simulink model "Shaber_GearShiftStrategy"  (R2023b)
settings: Solver=FixedStepAuto  StartTime=0.0  StopTime=inf  FixedStep=0.001  RelTol=1e-3
PreLoadFcn:
  | load('ACS_1DModel23_Parameters_v2.mat');
undefined symbols (not defined in the file): AmbTemp, CellContCur, G_A, Init_SoC, kI, kP, nP, nS, SoCmin, ThrottleBP, TMaxMotor, VehicleMass
libraries: nesl_utility x21, fl_lib x14, sdl_lib x8, simulink x3, autolibrcnetworksystem x1, autolibmappedmotorcommon x1, autolibshared x1
(part 2 of 2)

== system Shaber_GearShiftStrategy/Chassis/Subsystem2 ==
  Ideal Rotational Motion Sensor : fl_lib/Mechanical/Mechanical Sensors/Ideal Rotational Motion Sensor  reference=foundation.enum.MeasurementReference.difference  acceleration_port=false  velocity_port=true  position_port=true  wrap_angle=simscape.enum.onoff.off  offset=0 rad
  Ideal Torque Sensor : fl_lib/Mechanical/Mechanical Sensors/Ideal Torque Sensor
  Mechanical Rotational Reference1 : fl_lib/Mechanical/Rotational Elements/Mechanical Rotational Reference
  PS-Simulink Converter : nesl_utility/PS-Simulink Converter  PhysicalDomain=network_engine_domain  SubClassName=ps_output  LeftPortType=input  RightPortType=output  PseudoPeriodic=off  Frequencies=[]  VectorFormat=1-D array  Unit=N*m  AffineConversion=off
  PS-Simulink Converter1 : nesl_utility/PS-Simulink Converter  PhysicalDomain=network_engine_domain  SubClassName=ps_output  LeftPortType=input  RightPortType=output  PseudoPeriodic=off  Frequencies=[]  VectorFormat=1-D array  Unit=rpm  AffineConversion=off
  PS-Simulink Converter2 : nesl_utility/PS-Simulink Converter  PhysicalDomain=network_engine_domain  SubClassName=ps_output  LeftPortType=input  RightPortType=output  PseudoPeriodic=off  Frequencies=[]  VectorFormat=1-D array  Unit=1  AffineConversion=off
  Terminator2 : Terminator
  Terminator3 : Terminator
  Conn1 : PMIOPort  Side=Right
  Conn2 : PMIOPort  Port=2  Side=Left
  FW Spd : Outport
  wires:
  PS-Simulink Converter/1 -> Terminator3/1  "WheelFrTq"
  PS-Simulink Converter2/1 -> Terminator2/1  "WheelFrAcc"
  PS-Simulink Converter1/1 -> FW Spd/1  "FWSpd [rpm]"
  connections:
  Ideal Torque Sensor/LConn1 -- Conn2/RConn1
  Conn1/RConn1 -- Ideal Torque Sensor/RConn1 -- Ideal Rotational Motion Sensor/LConn1
  Mechanical Rotational Reference1/LConn1 -- Ideal Rotational Motion Sensor/RConn1
  PS-Simulink Converter1/LConn1 -- Ideal Rotational Motion Sensor/RConn2
  PS-Simulink Converter/LConn1 -- Ideal Torque Sensor/RConn2
  Ideal Rotational Motion Sensor/RConn3 -- PS-Simulink Converter2/LConn1

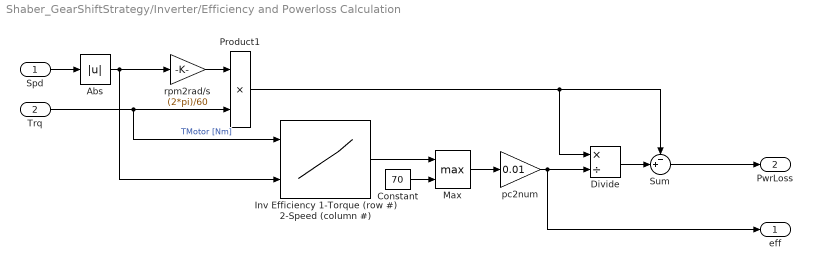
== system Shaber_GearShiftStrategy/Inverter/Efficiency and Powerloss Calculation ==
  Spd : Inport
  Trq : Inport  Port=2
  Abs : Abs  SaturateOnIntegerOverflow=off
  Constant : Constant  Value=70
  Divide : Product  Inputs=*/
  Inv Efficiency 1-Torque (row #) 2-Speed (column #) : Lookup_n-D  BreakpointsForDimension1=[-TMaxMotor TMaxMotor]  BreakpointsForDimension2=[0 7000]  Table=[0.8 0.9; 0.8 0.9]*100  InterpMethod=Cubic spline  ExtrapMethod=Cubic spline  InternalRulePriority=Speed  RndMeth=Simplest
      settings: InputPortMap=u0,u1
  Max : MinMax  Function=max  Inputs=2
  Product1 : Product
  Sum : Sum  Inputs=-+|
  pc2num : Gain  Gain=0.01
  rpm2rad/s : Gain  Gain=(2*pi)/60
  eff : Outport  VectorParamsAs1DForOutWhenUnconnected=off
  PwrLoss : Outport  Port=2  VectorParamsAs1DForOutWhenUnconnected=off
  wires:
  Product1/1 -> Sum/1, Divide/1
  Trq/1 -> Inv Efficiency 1-Torque (row #) 2-Speed (column #)/1, Product1/2  "TMotor [Nm]"
  Constant/1 -> Max/2
  Sum/1 -> PwrLoss/1
  Max/1 -> pc2num/1
  Divide/1 -> Sum/2
  rpm2rad/s/1 -> Product1/1
  Inv Efficiency 1-Torque (row #) 2-Speed (column #)/1 -> Max/1
  Spd/1 -> Abs/1
  Abs/1 -> rpm2rad/s/1, Inv Efficiency 1-Torque (row #) 2-Speed (column #)/2
  pc2num/1 -> Divide/2, eff/1

== system Shaber_GearShiftStrategy/Inverter/Transmission ==
  Abs1 : Abs  SaturateOnIntegerOverflow=off
  Constant : Constant  Value=2
  Data Type Conversion : DataTypeConversion  SaturateOnIntegerOverflow=off  RndMeth=Floor
  Relational Operator : RelationalOperator  Operator===  OutDataTypeStr=boolean  RndMeth=Simplest  InputSameDT=off
  Switch : Switch  Criteria=u2 > Threshold  SaturateOnIntegerOverflow=off  InputSameDT=off
  Transmission1 : Constant  Value=1*2.4*15/45
  Transmission2 : Constant  Value=1*1.5*15/45
  Transmission : Outport
  wires:
  [GearInd] -> Abs1/1
  Relational Operator/1 -> Data Type Conversion/1
  Transmission2/1 -> Switch/1
  Abs1/1 -> Relational Operator/2
  Switch/1 -> Transmission/1
  Constant/1 -> Relational Operator/1
  Transmission1/1 -> Switch/3
  Data Type Conversion/1 -> Switch/2

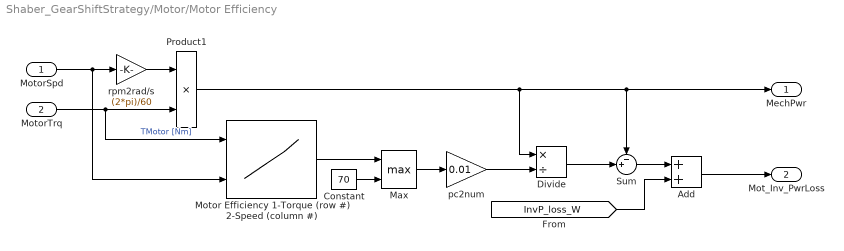
== system Shaber_GearShiftStrategy/Motor/Motor Efficiency ==
  MotorSpd : Inport
  MotorTrq : Inport  Port=2
  Add : Sum
  Constant : Constant  Value=70
  Divide : Product  Inputs=*/
  Max : MinMax  Function=max  Inputs=2
  Motor Efficiency 1-Torque (row #) 2-Speed (column #) : Lookup_n-D  BreakpointsForDimension1=[-TMaxMotor TMaxMotor]  BreakpointsForDimension2=[-7000 7000]  Table=[90 95; 90 95]  InterpMethod=Cubic spline  ExtrapMethod=Cubic spline  InternalRulePriority=Speed  RndMeth=Simplest
      settings: InputPortMap=u0,u1
  Product1 : Product
  Sum : Sum  Inputs=-+|
  pc2num : Gain  Gain=0.01
  rpm2rad/s : Gain  Gain=(2*pi)/60
  MechPwr : Outport  VectorParamsAs1DForOutWhenUnconnected=off
  Mot_Inv_PwrLoss : Outport  Port=2  VectorParamsAs1DForOutWhenUnconnected=off
  wires:
  Product1/1 -> MechPwr/1, Sum/1, Divide/1
  MotorTrq/1 -> Motor Efficiency 1-Torque (row #) 2-Speed (column #)/1, Product1/2  "TMotor [Nm]"
  Constant/1 -> Max/2
  Max/1 -> pc2num/1
  Divide/1 -> Sum/2
  rpm2rad/s/1 -> Product1/1
  MotorSpd/1 -> Motor Efficiency 1-Torque (row #) 2-Speed (column #)/2, rpm2rad/s/1
  Motor Efficiency 1-Torque (row #) 2-Speed (column #)/1 -> Max/1
  Sum/1 -> Add/1
  Add/1 -> Mot_Inv_PwrLoss/1
  [InvP_loss_W] -> Add/2
  pc2num/1 -> Divide/2

== system Shaber_GearShiftStrategy/Motor/Motor Time Constant (Response Smoothing) ==
  MaxT : Inport
  MotorTrqCmd : Inport  Port=2
  Divide2 : Product
  Gain : Gain  Gain=1/0.02
  Integrator : Integrator
  Interpolated Zero-crossing : Lookup_n-D  NumberOfTableDimensions=1  BreakpointsForDimension1=[-1 1]  Table=[-1 1]  ExtrapMethod=Clip  InternalRulePriority=Speed  RndMeth=Simplest
  Product1 : Product  Inputs=/*
  Sum : Sum  Inputs=|+-
  MotorTrq : Outport  InitialOutput=0  VectorParamsAs1DForOutWhenUnconnected=off
  wires:
  Sum/1 -> Integrator/1
  Gain/1 -> Product1/2, Sum/2
  Interpolated Zero-crossing/1 -> Divide2/2
  Integrator/1 -> Gain/1
  Divide2/1 -> MotorTrq/1
  MotorTrqCmd/1 -> Sum/1
  Product1/1 -> Interpolated Zero-crossing/1
  MaxT/1 -> Product1/1, Divide2/1

== system Shaber_GearShiftStrategy/Motor/Transmission ==
  Abs1 : Abs  SaturateOnIntegerOverflow=off
  Constant : Constant  Value=2
  Data Type Conversion : DataTypeConversion  SaturateOnIntegerOverflow=off  RndMeth=Floor
  Relational Operator : RelationalOperator  Operator===  OutDataTypeStr=boolean  RndMeth=Simplest  InputSameDT=off
  Switch : Switch  Criteria=u2 > Threshold  SaturateOnIntegerOverflow=off  InputSameDT=off
  Transmission1 : Constant  Value=1*2.4*15/45
  Transmission2 : Constant  Value=1*1.5*15/45
  Transmission : Outport
  wires:
  [GearInd] -> Abs1/1
  Relational Operator/1 -> Data Type Conversion/1
  Transmission2/1 -> Switch/1
  Abs1/1 -> Relational Operator/2
  Switch/1 -> Transmission/1
  Constant/1 -> Relational Operator/1
  Transmission1/1 -> Switch/3
  Data Type Conversion/1 -> Switch/2

== system Shaber_GearShiftStrategy/Rider/Subsystem1 ==
  Road Inclined (deg) : Inport
  Constant : Constant  Value=0
  Constant2 : Constant
  Display : Display
  Manual Switch : ManualSwitch
  Switch : Switch  Criteria=u2 > Threshold  SaturateOnIntegerOverflow=off  InputSameDT=off
  deg2rad : Gain  Gain=pi/180
  tag scope: RoadInclined=global
  wires:
  Manual Switch/1 -> Switch/1
  Constant/1 -> Manual Switch/2, Switch/3
  Switch/1 -> [RoadInclined]
  deg2rad/1 -> Display/1, Manual Switch/1  "rad"
  Constant2/1 -> Switch/2
  Road Inclined (deg)/1 -> deg2rad/1

== system Shaber_GearShiftStrategy/VSC/Checksum ==
  Torque_enable : Inport
  CurrentState : Inport  Port=2
  Driving State : Constant  Value=3
  Ignition State : Constant
  Logical Operator : Logic  AllPortsSameDT=off  OutDataTypeStr=boolean
  Logical Operator1 : Logic  AllPortsSameDT=off  OutDataTypeStr=boolean
  Logical Operator2 : Logic  AllPortsSameDT=off  OutDataTypeStr=boolean
  Out1 : Outport
  wires:
  Torque_enable/1 -> Logical Operator1/2
  Logical Operator2/1 -> Out1/1
  Ignition State/1 -> Logical Operator1/1
  CurrentState/1 -> Logical Operator/1
  Logical Operator/1 -> Logical Operator2/1
  Logical Operator1/1 -> Logical Operator2/2
  Driving State/1 -> Logical Operator/2

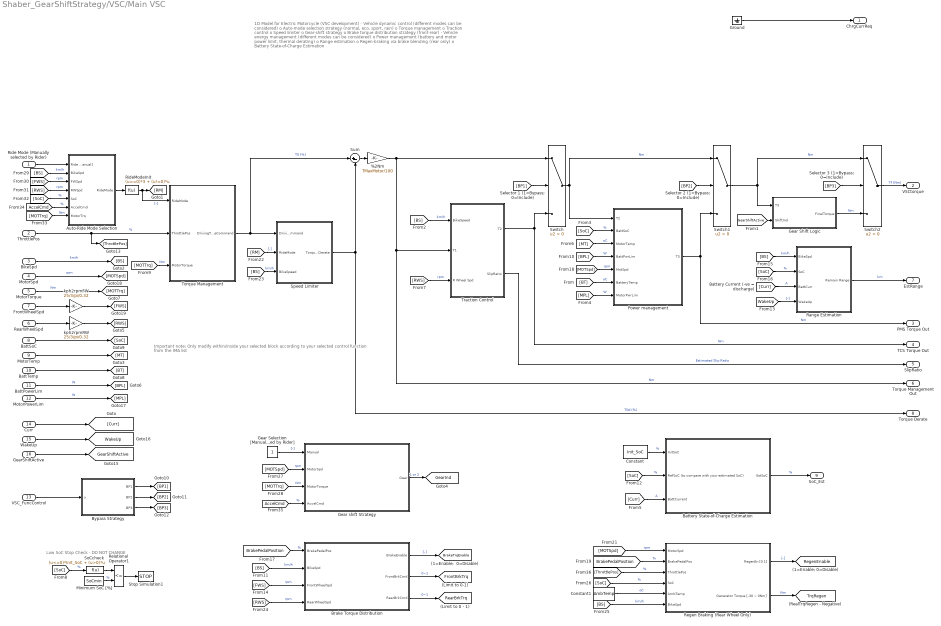
== system Shaber_GearShiftStrategy/VSC/Main VSC ==
  note: Low SoC Stop Check - DO NOT CHANGE
  note: 1D Model for Electric Motorcycle (VSC development)
      | · Vehicle dynamic control (different modes can be considered)
      | o Auto-mode selection strategy (normal, eco, sport, rain)
      | o Torque management
      | o Traction control
      | o Speed limiter
      | o Gear-shift strategy
      | o Brake torque distribution strategy (front-rear)
      | · Vehicle energy management (different modes can be considered)
      | o Power management (battery and motor power limit, thermal derating)
      | o Range estimation
      | o Regen-braking via brake blending (rear only)
      | o Battery State-of-Charge Estimation
  note: Important note:
      | Only modify within/inside your selected block according to your selected control function from the IMA list
  Ride Mode (Manually selected by Rider) : Inport
  ThrottlePos : Inport  Port=2
  BikeSpd : Inport  Port=3
  MotorSpd : Inport  Port=4
  MotorTorque : Inport  Port=5
  RearWheelSpd : Inport  Port=6
  FrontWheelSpd : Inport  Port=7
  BattSoC : Inport  Port=8
  MotorTemp : Inport  Port=9
  BattTemp : Inport  Port=10
  BattPowerLim : Inport  Port=11
  MotorPowerLim : Inport  Port=12
  VSC_FuncControl : Inport  Port=13
  Curr : Inport  Port=14
  WakeUp : Inport  Port=15
  GearShiftActive : Inport  Port=16
  %2Nm : Gain  Gain=TMaxMotor/100  OutDataTypeStr=Inherit: Same as input
  Auto-Ride Mode Selection : Subsystem
  Battery State-of-Charge Estimation : Subsystem
  Brake Torque Distribution : Subsystem
  Bypass Strategy : MATLAB Function  TreatAsAtomicUnit=on
  Constant : Constant  Value=Init_SoC
  Constant1 : Constant  Value=AmbTemp
  Gear Selection [Manually selected by Rider] : Constant
  Gear Shift Logic : Subsystem
  Gear shift Strategy : Subsystem
  Ground : Ground
  Minimum SoC [%] : Constant  Value=SoCmin
  Power management : Subsystem
  Range Estimation : Subsystem
  Regen Braking (Rear Wheel Only) : Subsystem
  Relational Operator1 : RelationalOperator  Operator=<=  OutDataTypeStr=boolean  RndMeth=Simplest  InputSameDT=off
  RideModeInit : Fcn  Expr=(u==0)*3 + (u!=0)*u
  SoCcheck : Fcn  Expr=(u<=0)*Init_SoC + (u>0)*u
  Speed Limiter : Subsystem
  Stop Simulation1 : Stop
  Sum : Sum  Inputs=|+-
  Switch : Switch  Criteria=u2 > Threshold  SaturateOnIntegerOverflow=off  InputSameDT=off
  Switch1 : Switch  Criteria=u2 > Threshold  SaturateOnIntegerOverflow=off  InputSameDT=off
  Switch2 : Switch  Criteria=u2 > Threshold  SaturateOnIntegerOverflow=off  InputSameDT=off
  Torque Management : Subsystem
  Traction Control : Subsystem
  kph2rpmFW : Gain  Gain=25/3/pi/0.32
  kph2rpmRW : Gain  Gain=25/3/pi/0.32
  ChrgCurrReq : Outport
  VSCtorque : Outport  Port=2
  PMS Torque Out : Outport  Port=3
  TCS Torque Out : Outport  Port=4
  SlipRatio : Outport  Port=5
  "Torque Management Out " : Outport  Port=6
  EstRange : Outport  Port=7
  Torque Derate : Outport  Port=8
  SoC_Est : Outport  Port=9
  tag scope: BrakeTrqEnable=global, FrontBrkTrq=global, GearInd=global, GearShiftActive=global, RearBrkTrq=global, RegenEnable=global, TrqRegen=global, WakeUp=global
  wires:
  Switch2/1 -> VSCtorque/1  "Tf (Nm)"
  [MOTSpd] -> Power management/5(MotSpd)  "rpm"
  BattPowerLim/1 -> [BPL]  "W"
  [BP2] -> Switch1/2
  BattSoC/1 -> [SoC]
  Bypass Strategy/1(BP1) -> [BP1]
  Ground/1 -> ChrgCurrReq/1
  RearWheelSpd/1 -> kph2rpmRW/1
  [BP3] -> Switch2/2
  FrontWheelSpd/1 -> kph2rpmFW/1
  [GearShiftActive] -> Gear Shift Logic/2(ShiftInd)
  [MPL] -> Power management/7(MotorPwrLim)  "W"
  BattTemp/1 -> [BT]
  [MT] -> Power management/3(MotorTemp)  "oC"
  Range Estimation/1(Remain Range) -> EstRange/1  "km"
  [BP1] -> Switch/2
  MotorPowerLim/1 -> [MPL]  "W"
  Traction Control/2(SlipRatio) -> SlipRatio/1  "Estimated Slip Ratio"
  [WakeUp] -> Range Estimation/4(WakeUp)  "[-]"
  Traction Control/1(T2) -> Switch/3, TCS Torque Out/1  "Nm"
  [Curr] -> Range Estimation/3(BattCurr)  "A"
  [BT] -> Power management/6(BatteryTemp)  "oC"
  GearShiftActive/1 -> [GearShiftActive]
  BikeSpd/1 -> [BS]  "km/h"
  ThrottlePos/1 -> [ThrottlePos], Torque Management/2(ThrottlePos)  "%"
  Power management/1(T3) -> PMS Torque Out/1, Switch1/3  "Nm"
  [BS] -> Range Estimation/1(BikeSpd)  "km/h"
  [SoC] -> Power management/2(BattSoC)  "%"
  [RWS] -> Traction Control/3(R Wheel Spd)  "rpm"
  kph2rpmRW/1 -> [RWS]
  kph2rpmFW/1 -> [FWS]
  Switch/1 -> Switch1/1, Power management/1(T2)  "Nm"
  [SoC] -> Range Estimation/2(SoC)  "%"
  VSC_FuncControl/1 -> Bypass Strategy/1(u)
  Switch1/1 -> Switch2/1, Gear Shift Logic/1(T3)  "Nm"
  MotorSpd/1 -> [MOTSpd]  "rpm"
  [BPL] -> Power management/4(BattPwrLim)  "W"
  Gear Shift Logic/1(FinalTorque) -> Switch2/3  "Nm"
  Curr/1 -> [Curr]
  RideModeInit/1 -> [RM], Torque Management/1(RideMode)  "[-]"
  Bypass Strategy/2(BP2) -> [BP2]
  WakeUp/1 -> [WakeUp]
  Bypass Strategy/3(BP3) -> [BP3]
  %2Nm/1 -> Switch/1, Traction Control/2(T1), "Torque Management Out "/1  "Nm"
  MotorTemp/1 -> [MT]
  Battery State-of-Charge Estimation/1(EstSoC) -> SoC_Est/1  "%"
  [Curr] -> Battery State-of-Charge Estimation/3(BattCurrent)  "A"
  Constant/1 -> Battery State-of-Charge Estimation/1(InitSoC)  "%"
  SoCcheck/1 -> Relational Operator1/1
  Minimum SoC [%]/1 -> Relational Operator1/2  "%"
  Relational Operator1/1 -> Stop Simulation1/1
  [SoC] -> SoCcheck/1  "%"
  Gear Selection [Manually selected by Rider]/1 -> Gear shift Strategy/1(Manual)  "[-]"
  Gear shift Strategy/1(Gear) -> [GearInd]  "1 or 2"
  MotorTorque/1 -> [MOTTrq]  "Nm"
  [MOTTrq] -> Torque Management/3(MotorTorque)  "Nm"
  [SoC] -> Battery State-of-Charge Estimation/2(RefSoC (to compare with your estimated SoC))  "%"
  Brake Torque Distribution/2(FrontBrkCmd) -> [FrontBrkTrq]  "0~1"
  Brake Torque Distribution/3(RearBrkCmd) -> [RearBrkTrq]  "0~1"
  [BrakePedalPosition] -> Brake Torque Distribution/1(BrakePedalPos)  "%"
  [BrakePedalPosition] -> Regen Braking (Rear Wheel Only)/2(BrakePedalPos)  "%"
  [ThrottlePos] -> Regen Braking (Rear Wheel Only)/3(ThrottlePos)  "%"
  Regen Braking (Rear Wheel Only)/1(RegenEn [0 1]) -> [RegenEnable]  "[-]"
  Regen Braking (Rear Wheel Only)/2(Generator Torque [-30 ~ 0Nm]) -> [TrqRegen]  "Nm"
  [MOTSpd] -> Regen Braking (Rear Wheel Only)/1(MotorSpd)  "rpm"
  Brake Torque Distribution/1(BrakeEnable) -> [BrakeTrqEnable]  "[-]"
  Sum/1 -> %2Nm/1
  Torque Management/1(DrivingTorqueCommand) -> Sum/1, Speed Limiter/1(DrivingTorqueCommand)  "T0 (%)"
  Speed Limiter/1("TorqueDerate ") -> Torque Derate/1, Sum/2  "T0d (%)"
  [RM] -> Speed Limiter/2(RideMode)  "[-]"
  [BS] -> Speed Limiter/3(BikeSpeed)  "km/h"
  [BS] -> Traction Control/1(BikeSpeed)  "km/h"
  [BS] -> Brake Torque Distribution/2(BikeSpd)  "km/h"
  [FWS] -> Brake Torque Distribution/3(FrontWheelSpd)  "rpm"
  [RWS] -> Brake Torque Distribution/4(RearWheelSpd)  "rpm"
  [BS] -> Regen Braking (Rear Wheel Only)/6(BikeSpd)  "km/h"
  [SoC] -> Regen Braking (Rear Wheel Only)/4(SoC)  "%"
  Constant1/1 -> Regen Braking (Rear Wheel Only)/5(AmbTemp)  "oC"
  [MOTSpd] -> Gear shift Strategy/2(MotorSpd)  "rpm"
  [MOTTrq] -> Gear shift Strategy/3(MotorTorque)  "Nm"
  [BS] -> Auto-Ride Mode Selection/2(BikeSpd)  "km/h"
  [FWS] -> Auto-Ride Mode Selection/3(FWSpd)  "rpm"
  [RWS] -> Auto-Ride Mode Selection/4(RWSpd)  "rpm"
  [SoC] -> Auto-Ride Mode Selection/5(SoC)  "%"
  [MOTTrq] -> Auto-Ride Mode Selection/7(MotorTrq)  "Nm"
  [AccelCmd] -> Auto-Ride Mode Selection/6(AccelCmd)  "%"
  [AccelCmd] -> Gear shift Strategy/4(AccelCmd)  "%"
  Ride Mode (Manually selected by Rider)/1 -> Auto-Ride Mode Selection/1(Ride Mode [Manual])
  Auto-Ride Mode Selection/1(RideMode) -> RideModeInit/1

== system Shaber_GearShiftStrategy/Chassis/2-Speeds CVT/Subsystem1 ==
  Ideal Rotational Motion Sensor : fl_lib/Mechanical/Mechanical Sensors/Ideal Rotational Motion Sensor  reference=foundation.enum.MeasurementReference.difference  acceleration_port=false  velocity_port=true  position_port=true  wrap_angle=simscape.enum.onoff.off  offset=0 rev
  Ideal Torque Sensor : fl_lib/Mechanical/Mechanical Sensors/Ideal Torque Sensor
  Mechanical Rotational Reference1 : fl_lib/Mechanical/Rotational Elements/Mechanical Rotational Reference
  PS-Simulink Converter : nesl_utility/PS-Simulink Converter  PhysicalDomain=network_engine_domain  SubClassName=ps_output  LeftPortType=input  RightPortType=output  PseudoPeriodic=off  Frequencies=[]  VectorFormat=1-D array  Unit=N*m  AffineConversion=off
  PS-Simulink Converter1 : nesl_utility/PS-Simulink Converter  PhysicalDomain=network_engine_domain  SubClassName=ps_output  LeftPortType=input  RightPortType=output  PseudoPeriodic=off  Frequencies=[]  VectorFormat=1-D array  Unit=rpm  AffineConversion=off
  PS-Simulink Converter2 : nesl_utility/PS-Simulink Converter  PhysicalDomain=network_engine_domain  SubClassName=ps_output  LeftPortType=input  RightPortType=output  PseudoPeriodic=off  Frequencies=[]  VectorFormat=1-D array  Unit=1  AffineConversion=off
  Terminator2 : Terminator
  Conn1 : PMIOPort  Side=Right
  Conn2 : PMIOPort  Port=2  Side=Left
  Spd : Outport
  Trq : Outport  Port=2
  wires:
  PS-Simulink Converter2/1 -> Terminator2/1  "OutShaftAcc"
  PS-Simulink Converter/1 -> Trq/1  "OutShaftTq"
  PS-Simulink Converter1/1 -> Spd/1  "OutShaftSpd(rpm)"
  connections:
  Ideal Rotational Motion Sensor/RConn3 -- PS-Simulink Converter2/LConn1
  PS-Simulink Converter/LConn1 -- Ideal Torque Sensor/RConn2
  PS-Simulink Converter1/LConn1 -- Ideal Rotational Motion Sensor/RConn2
  Mechanical Rotational Reference1/LConn1 -- Ideal Rotational Motion Sensor/RConn1
  Conn1/RConn1 -- Ideal Rotational Motion Sensor/LConn1 -- Ideal Torque Sensor/RConn1
  Ideal Torque Sensor/LConn1 -- Conn2/RConn1

== system Shaber_GearShiftStrategy/VSC/Main VSC/Auto-Ride Mode Selection ==
  note: To be replaced by your logic
  note: Ride Mode definition: 1 = Rain ; 2 = Eco ; 3 = Normal ; 4 = Sport
      |
      | Requirement:
      | - Develop a logic in Stateflow to decide the bike operational mode according to the update of system state (inputs available for this function)
      |
      | Example: Switch to Sport mode when having high AccelCmd
      |
      | Inputs:
      | - BikeSpd, FWSpd, RWSpd, SoC, AccelCmd, MotorTrq
  Ride Mode [Manual] : Inport
  BikeSpd : Inport  Port=2
  FWSpd : Inport  Port=3
  RWSpd : Inport  Port=4
  SoC : Inport  Port=5
  AccelCmd : Inport  Port=6
  MotorTrq : Inport  Port=7
  Constant : Constant  Value=0
  Ground : Ground
  Switch : Switch  Criteria=u2 > Threshold  SaturateOnIntegerOverflow=off  InputSameDT=off
  RideMode : Outport
  wires:
  Ride Mode [Manual]/1 -> Switch/3  "Manual"
  Switch/1 -> RideMode/1
  Constant/1 -> Switch/2
  Ground/1 -> Switch/1

== system Shaber_GearShiftStrategy/VSC/Main VSC/Battery State-of-Charge Estimation ==
  note: Requirement:
      | Create a logic to estimate the State of Charge of the battery:
      | - Use any input from the MainBus
      | - Build an Equivalent Circuit Model (ECM) using Simulink blocks (not using battery components in Simulink)
      | - Limit the SoC within 0 - 100%
      | - Employ the InitSoC input as the initial SoC of the battery (can be used to interpolate the Initial remained Capacity)
      |
      | Note: can get ECM parameters from the "Battery Pack" block
  InitSoC : Inport
  RefSoC (to compare with your estimated SoC) : Inport  Port=2
  BattCurrent : Inport  Port=3
  EstSoC : Outport

== system Shaber_GearShiftStrategy/VSC/Main VSC/Brake Torque Distribution ==
  note: BrakeEnable = 0: use default values defined from the model (Front/Rear = 20%/80% by default)
      | BrakeEnable = 1: use your own brake torque distribution
  note: Requirement:
      | Develop a controller to distribute the brake torque applied to the front and rear wheels (already added in the Chassis model) when applying Brake
      |
      | Note:
      | use any input from the Bus or elsewhere
      |
      | Example: some ideas about brake torque distribution from this link:
      |
      | https://www.drivingtests.co.nz/roadcode-questions/motorbike/motorbike-specific-questions/how-much-braking-comes-from-the-front-wh/
      |
      | https://www.lazymotorbike.eu/tips/braking/
  BrakePedalPos : Inport
  BikeSpd : Inport  Port=2
  FrontWheelSpd : Inport  Port=3
  RearWheelSpd : Inport  Port=4
  Ground : Ground
  Terminator : Terminator
  km/h 2 rpm : Gain  Gain=25/3/pi/0.32
  BrakeEnable : Outport
  FrontBrkCmd : Outport  Port=2
  RearBrkCmd : Outport  Port=3
  wires:
  Ground/1 -> BrakeEnable/1
  BikeSpd/1 -> km/h 2 rpm/1  "km/h"
  km/h 2 rpm/1 -> Terminator/1  "rpm"

== system Shaber_GearShiftStrategy/VSC/Main VSC/Gear Shift Logic ==
  note: Gear Shift Logic - DO NOT TOUCH
  T3 : Inport
  ShiftInd : Inport  Port=2
  Gear Shift Logic : Stateflow chart  TreatAsAtomicUnit=on
  Sum : Sum  Inputs=|+-
  FinalTorque : Outport
  wires:
  Gear Shift Logic/1(TqMod) -> Sum/2
  ShiftInd/1 -> Gear Shift Logic/2(ShiftInd)
  T3/1 -> Sum/1, Gear Shift Logic/1(T3)
  Sum/1 -> FinalTorque/1

== system Shaber_GearShiftStrategy/VSC/Main VSC/Gear shift Strategy ==
  note: Gear 1 ratio = 2.5 (speed reduction)
      | Gear 2 ratio = 4 (speed reduction)
      |
      | Requirement:
      | Develop a logic to switch between 2 speeds of the CVT transmission as shown in the Chassis model (can be expanded to more than 2 ratios). The logic could be based on vehicle speed, motor speed, Acceleration command, motor torque ...
      |
      | Example:
      | when high MotorTorque, Gear 2 can be used to increase Torque;
      | when high AccelCmd and low MotorTorque, Gear 1 can be used.
  Manual : Inport
  MotorSpd : Inport  Port=2
  MotorTorque : Inport  Port=3
  AccelCmd : Inport  Port=4
  Bus Selector : BusSelector  OutputSignals=RiderCmd.RiderMode
  Chart : Stateflow chart  TreatAsAtomicUnit=on
  Scope : Scope  NumInputPorts=3
  Gear : Outport
  wires:
  [BUS] -> Bus Selector/1
  AccelCmd/1 -> Chart/3(AccelCmd), Scope/2
  Bus Selector/1 -> Chart/4(RiderMode)  "<RiderMode>"
  Manual/1 -> Chart/1(Manual)
  Chart/1(Gear) -> Gear/1, Scope/3
  MotorSpd/1 -> Chart/2(MotorSpd), Scope/1

== system Shaber_GearShiftStrategy/VSC/Main VSC/Power management ==
  note: Requirement:
      | Develop the following logics:
      | - Battery power limit (using BattSoC, BattPwrLim)
      | - Motor power limit (using MotorPwrLim)
      | - Thermal derating (using MotorTemp and BatteryTemp)
      |
      | Note: T3 = T2 - T2d
      | BattPwrLim and MotorPwrLim are the maximum power available on Battery and Motor, respectively
      |
      | Example:
      | when high MotorTemp or BatteryTemp, Torque output will be derated
  T2 : Inport
  BattSoC : Inport  Port=2
  MotorTemp : Inport  Port=3
  BattPwrLim : Inport  Port=4
  MotSpd : Inport  Port=5
  BatteryTemp : Inport  Port=6
  MotorPwrLim : Inport  Port=7
  Ground : Ground
  Sum : Sum  Inputs=-+|
  T3 : Outport
  wires:
  T2/1 -> Sum/2
  Sum/1 -> T3/1
  Ground/1 -> Sum/1  "T2d (Nm)"

== system Shaber_GearShiftStrategy/VSC/Main VSC/Range Estimation ==
  BikeSpd : Inport
  SoC : Inport  Port=2
  BattCurr : Inport  Port=3
  WakeUp : Inport  Port=4
  AmbTemp : Constant  Value=AmbTemp
  Minimum Allowable Battery SoC [%] : Constant  Value=SoCmin
  Model Discrete Sample Time [s] : Constant  Value=0.01
  Range estimation : Subsystem
  SoCcheck : Fcn  Expr=(u<=0)*Init_SoC + (u>0)*u
  Theoretical Max. Range [km] : Constant  Value=150
  Typical Consumption Rate [%/km] : Constant  Value=0.625
  Remain Range : Outport
  wires:
  Range estimation/1(Ro) -> Remain Range/1  "km"
  Minimum Allowable Battery SoC [%]/1 -> Range estimation/4(SoCmin)  "%"
  AmbTemp/1 -> Range estimation/8(AmbTemp)  "oC"
  SoCcheck/1 -> Range estimation/5(SoC)  "%"
  BattCurr/1 -> Range estimation/7(BattCurr)  "A"
  SoC/1 -> SoCcheck/1
  Typical Consumption Rate [%/km]/1 -> Range estimation/6(AvgConR)  "%SoC/km"
  Model Discrete Sample Time [s]/1 -> Range estimation/2(dT)  "s"
  BikeSpd/1 -> Range estimation/1(BSpd)  "km/h"
  WakeUp/1 -> Range estimation/9(WakeUp)  "on/off"
  Theoretical Max. Range [km]/1 -> Range estimation/3(RMax)  "km"

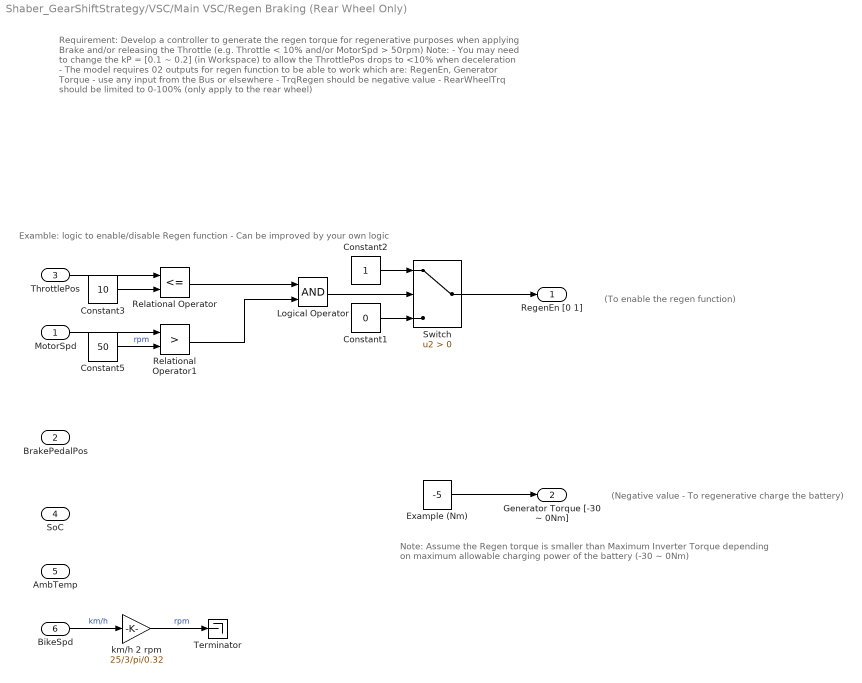
== system Shaber_GearShiftStrategy/VSC/Main VSC/Regen Braking (Rear Wheel Only) ==
  note: Examble: logic to enable/disable Regen function - Can be improved by your own logic
  note: (To enable the regen function)
  note: (Negative value - To regenerative charge the battery)
  note: Requirement:
      | Develop a controller to generate the regen torque for regenerative purposes when applying Brake and/or releasing the Throttle (e.g. Throttle < 10% and/or MotorSpd > 50rpm)
      |
      | Note:
      | - You may need to change the kP = [0.1 ~ 0.2] (in Workspace) to allow the ThrottlePos drops to <10% when deceleration
      | - The model requires 02 outputs for regen function to be able to work which are: RegenEn, Generator Torque
      | - use any input from the Bus or elsewhere
      | - TrqRegen should be negative value
      | - RearWheelTrq should be limited to 0-100% (only apply to the rear wheel)
  note: Note: Assume the Regen torque is smaller than Maximum Inverter Torque
      | depending on maximum allowable charging power of the battery
      | (-30 ~ 0Nm)
  MotorSpd : Inport
  BrakePedalPos : Inport  Port=2
  ThrottlePos : Inport  Port=3
  SoC : Inport  Port=4
  AmbTemp : Inport  Port=5
  BikeSpd : Inport  Port=6
  Constant1 : Constant  Value=0
  Constant2 : Constant
  Constant3 : Constant  Value=10
  Constant5 : Constant  Value=50
  Example (Nm) : Constant  Value=-5
  Logical Operator : Logic  AllPortsSameDT=off  OutDataTypeStr=boolean
  Relational Operator : RelationalOperator  Operator=<=  OutDataTypeStr=boolean  RndMeth=Simplest  InputSameDT=off
  Relational Operator1 : RelationalOperator  Operator=>  OutDataTypeStr=boolean  RndMeth=Simplest  InputSameDT=off
  Switch : Switch  Criteria=u2 > Threshold  SaturateOnIntegerOverflow=off  InputSameDT=off
  Terminator : Terminator
  km/h 2 rpm : Gain  Gain=25/3/pi/0.32
  RegenEn [0 1] : Outport
  Generator Torque [-30 ~ 0Nm] : Outport  Port=2
  wires:
  Example (Nm)/1 -> Generator Torque [-30 ~ 0Nm]/1
  Switch/1 -> RegenEn [0 1]/1
  Constant1/1 -> Switch/3
  Constant2/1 -> Switch/1
  Logical Operator/1 -> Switch/2
  ThrottlePos/1 -> Relational Operator/1
  Constant3/1 -> Relational Operator/2
  MotorSpd/1 -> Relational Operator1/1
  Constant5/1 -> Relational Operator1/2  "rpm"
  Relational Operator/1 -> Logical Operator/1
  Relational Operator1/1 -> Logical Operator/2
  km/h 2 rpm/1 -> Terminator/1  "rpm"
  BikeSpd/1 -> km/h 2 rpm/1  "km/h"

== system Shaber_GearShiftStrategy/VSC/Main VSC/Speed Limiter ==
  note: Fixed saturation - DO NOT CHANGE
  note: Requirement:
      | Create a closed-loop controller inside "Forward Torque Derater" block to ensure that the bike speed does not come out of range within its current operation mode, by considering:
      | Input: (you can use all or some of these available inputs: BikeSpeed, RideMode, TorqueDemand), more inputs can be collected from the Bus
      | Output: controlled TorqueDerate
      | Note: the logic inside "Forward Torque Derater" block is an example using open-loop control to generate the TorqueDerate
  DrivingTorqueCommand : Inport
  RideMode : Inport  Port=2
  BikeSpeed : Inport  Port=3
  Constant1 : Constant  Value=0
  Forward Torque Derater : Subsystem
  Saturation : Saturate  UpperLimit=TMaxMotor  LowerLimit=0
  Saturation Dynamic : simulink/Discontinuities/Saturation Dynamic  OutMin=[]  OutMax=[]  OutDataTypeStr=Inherit: Same as second input  OutDataType=fixdt(1, 16)  OutScaling=2^-10  DoSatur=off
  "TorqueDerate " : Outport
  wires:
  Saturation Dynamic/1 -> "TorqueDerate "/1  "T0d"
  RideMode/1 -> Forward Torque Derater/1(RideMode)
  BikeSpeed/1 -> Forward Torque Derater/2(BikeSpeed)  "km/h"
  Constant1/1 -> Saturation Dynamic/3
  Forward Torque Derater/1(TqMod) -> Saturation Dynamic/2
  DrivingTorqueCommand/1 -> Saturation/1
  Saturation/1 -> Saturation Dynamic/1

== system Shaber_GearShiftStrategy/VSC/Main VSC/Torque Management ==
  note: y is the Reference Torque for your closed-loop controller
  note: Fixed Open-loop Torque Map - DO NOT CHANGE or DELETE
  note: Requirement:
      |
      | Create a closed-loop controller to control the torque demand (TqDemand) to follow the desired torque (y) interpolated based on ThrottleBP position
      | - Use MotorTorque input as the actual torque feedback of the motor
      |
      | Note: in here we have an open-loop torque demand (y), which is linear interpolated based on the ThrottleBP and RideMode
  RideMode : Inport
  ThrottlePos : Inport  Port=2
  MotorTorque : Inport  Port=3
  Constant1 : Constant  Value=ThrottleBP  VectorParams1D=off
  Eco : Constant  Value=[0 0 0 4 8 13 16 20 25 30 35 40 45 48 50 55 60 65 70 75 80]'  VectorParams1D=off
  Linear interpolation : simulink/Lookup Tables/Lookup Table Dynamic  LookUpMeth=Interpolation-Use End Values  OutDataType=fixdt('double')  OutScaling=[]  OutputDataTypeScalingMode=Specify via dialog  OutDataTypeStr=double  DoSatur=off
  Multiport Switch : MultiPortSwitch  Inputs=4  DataPortForDefault=Additional data port  SaturateOnIntegerOverflow=off  InputSameDT=off
  Norm : Constant  Value=[0 0 0 5 10 15 20 28 35 40 45 50 55 60 65 70 80 85 90 95 100]'  VectorParams1D=off
  Rain : Constant  Value=[0 0 0 3 8 13 18 22 28 32 36 40 44 48 52 56 60 64 66 68 70]'  VectorParams1D=off
  Sport : Constant  Value=[0 0 0 5 15 20 25 30 40 50 55 60 65 75 80 90 95 100 100 100 100]'  VectorParams1D=off
  DrivingTorqueCommand : Outport
  wires:
  RideMode/1 -> Multiport Switch/1
  Constant1/1 -> Linear interpolation/2
  Multiport Switch/1 -> Linear interpolation/3
  Rain/1 -> Multiport Switch/2  "Rain"
  Eco/1 -> Multiport Switch/3  "Eco"
  Norm/1 -> Multiport Switch/6, Multiport Switch/4  "Norm"
  ThrottlePos/1 -> Linear interpolation/1
  Sport/1 -> Multiport Switch/5  "Sport"
  Linear interpolation/1 -> DrivingTorqueCommand/1

== system Shaber_GearShiftStrategy/VSC/Main VSC/Traction Control ==
  note: Requirement:
      | Develop a logic for Traction control derater
      | - Calculate SlipRatio using Front and Rear wheel speeds
      | - A logic to define the Traction control derater for T1d (to reduce the wheel slip when operating at different road conditions)
      |
      | Note: T2 = T1 - T1d
  BikeSpeed : Inport
  T1 : Inport  Port=2  OutDataTypeStr=double
  R Wheel Spd : Inport  Port=3
  Ground : Ground
  Sum : Sum  Inputs=-+|
  Terminator : Terminator
  Terminator1 : Terminator
  Traction Control Derater : Subsystem
  km/h2rpm : Gain  Gain=25/3/pi/0.32
  T2 : Outport
  SlipRatio : Outport  Port=2
  wires:
  Traction Control Derater/1(T1d) -> Sum/1  "Nm"
  T1/1 -> Sum/2, Traction Control Derater/1(T1)
  Sum/1 -> T2/1
  R Wheel Spd/1 -> Terminator/1  "rpm"
  BikeSpeed/1 -> km/h2rpm/1  "km/h"
  Ground/1 -> SlipRatio/1
  km/h2rpm/1 -> Terminator1/1  "rpm"

== system Shaber_GearShiftStrategy/VSC/Main VSC/Range Estimation/Range estimation ==
  note: Requirement:
      | Develop a logic to estimate the remaining range of the bike
      | - Use any inputs provided here
      | - other inputs can be collected from Bus
      |
      | Note:
      | - initial remaining range could be interpolated based on current SoC
      | - estimated range should be then derived based on several inputs, such as SOC, actual travel distance (integration of bikespeed), actual SOC drop rate
      | - WakeUp signal is to start the process/update
  BSpd : Inport
  dT : Inport  Port=2
  RMax : Inport  Port=3
  SoCmin : Inport  Port=4
  SoC : Inport  Port=5
  AvgConR : Inport  Port=6
  BattCurr : Inport  Port=7
  AmbTemp : Inport  Port=8
  WakeUp : Inport  Port=9
  Constant : Constant  Value=0
  Ro : Outport
  wires:
  Constant/1 -> Ro/1

== system Shaber_GearShiftStrategy/VSC/Main VSC/Speed Limiter/Forward Torque Derater ==
  note: RAIN
  note: ECO
  note: NORMAL
  note: SPORT
  note: NORMAL (Default)
  RideMode : Inport
  BikeSpeed : Inport  Port=2
  1-D Lookup Table : Lookup_n-D  NumberOfTableDimensions=1  BreakpointsForDimension1=[0,112,114,116,119,120,120.5,121,150]  Table=[0,0,0,2,15,25,35,45,70]*TMaxMotor/100  InternalRulePriority=Speed  RndMeth=Simplest
  1-D Lookup Table2 : Lookup_n-D  NumberOfTableDimensions=1  BreakpointsForDimension1=[0,112,114,116,119,120,120.5,121,150]  Table=[0,0,0,2,15,25,35,45,70]*TMaxMotor/100  InternalRulePriority=Speed  RndMeth=Simplest
  1-D Lookup Table4 : Lookup_n-D  NumberOfTableDimensions=1  BreakpointsForDimension1=[0,137,139,142,144,145,145.5,146,170]  Table=[0,0,0,0,10,21,28,34,100]*TMaxMotor/100  InternalRulePriority=Speed  RndMeth=Simplest
  1-D Lookup Table6 : Lookup_n-D  NumberOfTableDimensions=1  BreakpointsForDimension1=[0,177,179,181,183,184,185,185.5,186,200]  Table=[0,0,0,0,0,0,2,5,10,20]*TMaxMotor/100  InternalRulePriority=Speed  RndMeth=Simplest
  1-D Lookup Table8 : Lookup_n-D  NumberOfTableDimensions=1  BreakpointsForDimension1=[0,137,139,142,144,145,145.5,146,170]  Table=[0,0,0,0,10,21,28,34,100]*TMaxMotor/100  InternalRulePriority=Speed  RndMeth=Simplest
  Multiport Switch : MultiPortSwitch  Inputs=4  DataPortForDefault=Additional data port  DiagnosticForDefault=None  SaturateOnIntegerOverflow=off  InputSameDT=off
  TqMod : Outport
  wires:
  1-D Lookup Table8/1 -> Multiport Switch/6
  1-D Lookup Table6/1 -> Multiport Switch/5
  BikeSpeed/1 -> 1-D Lookup Table8/1, 1-D Lookup Table6/1, 1-D Lookup Table4/1, 1-D Lookup Table2/1, 1-D Lookup Table/1
  1-D Lookup Table/1 -> Multiport Switch/2
  1-D Lookup Table2/1 -> Multiport Switch/3
  1-D Lookup Table4/1 -> Multiport Switch/4
  RideMode/1 -> Multiport Switch/1
  Multiport Switch/1 -> TqMod/1

== system Shaber_GearShiftStrategy/VSC/Main VSC/Traction Control/Traction Control Derater ==
  T1 : Inport
  Ground : Ground
  Terminator : Terminator
  T1d : Outport
  wires:
  Ground/1 -> T1d/1
  T1/1 -> Terminator/1

== stateflow chart Shaber_GearShiftStrategy/VSC/Main VSC/Gear shift Strategy/Chart ==
  settings: executeAtInitialization=1
  state Gear2
    entry:
    Gear = 2;
    if (RiderMode >= 1 && RiderMode <= 4)
    upRPM = upRPM_table(RiderMode);
    dnRPM = dnRPM_table(RiderMode);
    kd    = kd_table(RiderMode);
    end
    during:
    if (RiderMode >= 1 && RiderMode <= 4)
    upRPM = upRPM_table(RiderMode);
    dnRPM = dnRPM_table(RiderMode);
    kd    = kd_table(RiderMode);
    end
  state Gear1
    entry:
    Gear = 1;
    if (RiderMode >= 1 && RiderMode <= 4)
    upRPM = upRPM_table(RiderMode);
    dnRPM = dnRPM_table(RiderMode);
    kd    = kd_table(RiderMode);
    end
    during:
    if (RiderMode >= 1 && RiderMode <= 4)
    upRPM = upRPM_table(RiderMode);
    dnRPM = dnRPM_table(RiderMode);
    kd    = kd_table(RiderMode);
    end
  (default) -> (junction 52)
  (junction 52) -> Gear1 [order 2] : [Manual == 1]
  (junction 52) -> Gear2 [order 1]
  Gear1 -> Gear2 : [MotorSpd < dnRPM || AccelCmd > kd]
  Gear2 -> Gear1 : [MotorSpd > upRPM && AccelCmd <= kd]
  data: Manual input double; MotorSpd input double; AccelCmd input double; RiderMode input double; Gear output double =2; dnRPM local double =0; kd local double =0; upRPM local double =0; upRPM_table local double size=[1, 4] =[80, 100, 120, 140]; dnRPM_table local double size=[1, 4] =[50, 65, 80, 100]; kd_table local double size=[1, 4] =[100, 34, 30, 24]

== matlab function Shaber_GearShiftStrategy/VSC/Main VSC/Bypass Strategy ==
  data: u input; BP1 output; BP2 output; BP3 output
function [BP1, BP2, BP3] = fcn(u)
%By pass condition to include WMG VSC control features
if u == 1       %Only Torque control included
    BP1 = 1;
    BP2 = 1;
    BP3 = 1;
elseif u == 2   %Only Torque and Traction control included
    BP1 = 0;
    BP2 = 1;
    BP3 = 1;
elseif u == 3   %Only Torque, Traction and Power management included
    BP1 = 0;
    BP2 = 0;
    BP3 = 1;
else            %All 4 features included
    BP1 = 0;
    BP2 = 0;
    BP3 = 0;
end

== stateflow chart Shaber_GearShiftStrategy/VSC/Main VSC/Gear Shift Logic/Gear Shift Logic ==
  state Waiting
    entry:
    TqMod = 0;
    during:
    TqMod = 0;
  state Shifting
    entry:
    TqMod = T3;
    during:
    TqMod = T3;
  (default) -> Waiting
  Waiting -> Shifting : [ShiftInd == 1]
  Shifting -> Waiting : [ShiftInd == 0]
  data: TqMod output; T3 input; ShiftInd input

== matlab function Shaber_GearShiftStrategy/Rider/MATLAB Function ==
  data: clock input; Ignition_sw output; SideStand_sw output; Brake_sw output; AccPed_pc output; Run_sw output; ChargerCnnt output; Start_sw output
function [Ignition_sw, SideStand_sw, Brake_sw, AccPed_pc, Run_sw, ChargerCnnt, Start_sw] = fcn(clock)

    if clock < 2   %first 2 seconds: bike's parking and charging
        Ignition_sw = 0;
        SideStand_sw = 1;
        Brake_sw = 0;
        AccPed_pc = 0;
        Run_sw = 0;
        ChargerCnnt = 1;
        Start_sw = 0;
    elseif clock <= 3   %from 2nd to 3rd second: battery unplugged and ignition ON (State 1), 
        %pause 2 seconds in Ingition mode (this mode)
        Ignition_sw = 1;
        SideStand_sw = 1;
        Brake_sw = 0;
        AccPed_pc = 0;
        Run_sw = 0;
        ChargerCnnt = 0;
        Start_sw = 0;
    elseif clock <= 5.1   %from 3rd to 5th second: Crank ON (State 2)
        Ignition_sw = 1;
        SideStand_sw = 0;
        Brake_sw = 1;
        AccPed_pc = 0;
        Run_sw = 1;
        ChargerCnnt = 0;
        Start_sw = 1;
    else        %Bike will run after 5.1 second
        Ignition_sw = 1;
        SideStand_sw = 0;
        Brake_sw = 0;
        AccPed_pc = 0;
        Run_sw = 1;
        ChargerCnnt = 0;
        Start_sw = 0;
    end
 
end

== stateflow chart Shaber_GearShiftStrategy/VSC/VSC High Level StateMachine ==
  state OFF
    entry:
    CurrentState = 0;
    Torque_enable = 0;
    state Shutdown
    state Wake_Up
      entry:
      WakeUp_Status = 1;
    (default) -> Shutdown
    Shutdown -> Wake_Up : [Ign_switch == 1]
    Wake_Up -> (junction 86) [order 2]
  state Charging
    entry:
    CurrentState = 4;
    Torque_enable = 0;
    state Charging_ON
    state Charging_OFF
    (default) -> Charging_ON
    Charging_ON -> Charging_OFF : [Ign_switch == 1]
    Charging_OFF -> Charging_ON : [Ign_switch == 0]
  note: CurrentState : OFF = 0, Ignition_ON = 1, Crank = 2, Drive_Ready = 3, Charging = 4
  state Ignition_ON
    entry:
    CurrentState = 1;
    Torque_enable = 0;
  state Crank
    entry:
    CurrentState = 2;
    Torque_enable = 0;
    during:
    HVBattContactorReq = 1;
  state Drive_Ready
    entry:
    CurrentState = 3;
    Torque_enable = 1;
  (default) -> OFF
  Charging -> Shutdown : [ ChargerConnect == 0 ]
  (junction 53) -> Shutdown
  Wake_Up -> Ignition_ON [order 1] : [(ChargerConnect == 0) && ...
      |  (Ign_switch == 1) && ...
      |  (WakeUp_Status == 1)]
  (junction 86) -> Charging : [WakeUp_Status == 1&&ChargerConnect == 1 &&...
      |  VehSpd_kph == 0 && Ign_switch == 0]
  (junction 51) -> (junction 53)
  (junction 49) -> (junction 51) : [(Ign_switch == 0&&VehSpd_kph == 0&&AccPed_pc == 0)]
      | {Torque_enable = 0;}
  Ignition_ON -> (junction 53) [order 1] : [Ign_switch == 0]
  Ignition_ON -> Crank [order 2] : [(AccPed_pc == 0) && (Brake_switch == 1) && ...
      | (duration(Start_switch == 1)>1)]
  Crank -> Ignition_ON [order 2] : [duration(HVBattContactorStatus == 0)>5 ]
  Crank -> Drive_Ready [order 1] : [HVBattContactorStatus == 1]
  Drive_Ready -> (junction 49)
  data: Ign_switch input; Brake_switch input; AccPed_pc input; ChargerConnect input; Ignition_ON constant double =1; Charging constant double =4; HVBattContactorReq output; HVBattContactorStatus input; Drive_Ready constant double =3; Crank constant double =2; VehSpd_kph input; Torque_enable output; Wakeup_request local; WakeUp_Status local =0; Start_switch input; CurrentState output
